simulink model "prueba_dynamixel"  (R2020b)
settings: Solver=VariableStepAuto  StartTime=0.0  StopTime=10.0  RelTol=1e-3
values from neighbouring files (symbols this model uses):
  ADDR_MX_GOAL_POSITION = 30    [variables_dynamixel.m]
  ADDR_MX_PRESENT_POSITION = 36    [variables_dynamixel.m]
  ADDR_MX_TORQUE_ENABLE = 24    [variables_dynamixel.m]
  baud_rate = 57600    [variables_dynamixel.m]
  dynamixel_id = 1    [variables_dynamixel.m]
  protocol_version = 1    [variables_dynamixel.m]
settings Model: Creator=johnc  LastModifiedBy=johnc

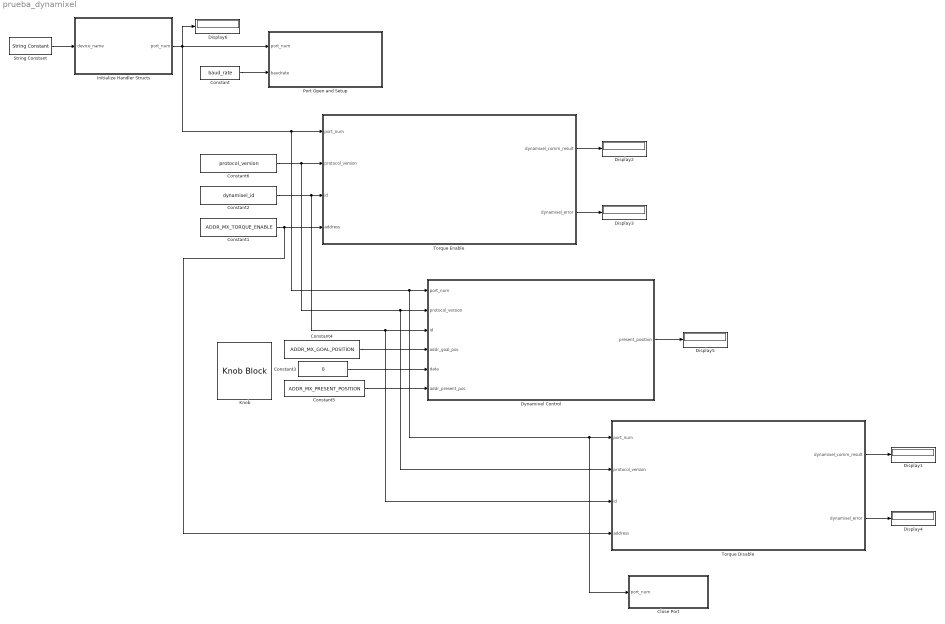
== system prueba_dynamixel ==
  Close Port : MATLAB Function  TreatAsAtomicUnit=on
  Constant : Constant  Value=baud_rate
  Constant1 : Constant  Value=ADDR_MX_TORQUE_ENABLE
  Constant2 : Constant  Value=dynamixel_id
  Constant3 : Constant  Value=0
  Constant4 : Constant  Value=ADDR_MX_GOAL_POSITION
  Constant5 : Constant  Value=ADDR_MX_PRESENT_POSITION
  Constant6 : Constant  Value=protocol_version
  Display{1..6} (6 alike) : Display
  Dynamixel Control : Subsystem
  Initialize Handler Structs : Subsystem
  Knob : KnobBlock  ScaleMax=1023
  Port Open and Setup : Subsystem
  String Constant : StringConstant  String=device_name
  Torque Disable : Subsystem
  Torque Enable : Subsystem
  wires:
  Torque Enable/1(dynamixel_comm_result) -> Display2/1
  Torque Enable/2(dynamixel_error) -> Display3/1
  String Constant/1 -> Initialize Handler Structs/1(device_name)
  Initialize Handler Structs/1(port_num) -> Close Port/1(port_num), Torque Disable/1(port_num), Dynamixel Control/1(port_num), Torque Enable/1(port_num), Display6/1, Port Open and Setup/1(port_num)
  Constant/1 -> Port Open and Setup/2(baudrate)
  Constant1/1 -> Torque Enable/4(address), Torque Disable/4(address)
  Constant2/1 -> Torque Disable/3(id), Dynamixel Control/3(id), Torque Enable/3(id)
  Torque Disable/1(dynamixel_comm_result) -> Display1/1
  Torque Disable/2(dynamixel_error) -> Display4/1
  Dynamixel Control/1(present_position) -> Display5/1
  Constant3/1 -> Dynamixel Control/5(data)
  Constant5/1 -> Dynamixel Control/6(addr_present_pos)
  Constant4/1 -> Dynamixel Control/4(addr_goal_pos)
  Constant6/1 -> Torque Disable/2(protocol_version), Dynamixel Control/2(protocol_version), Torque Enable/2(protocol_version)

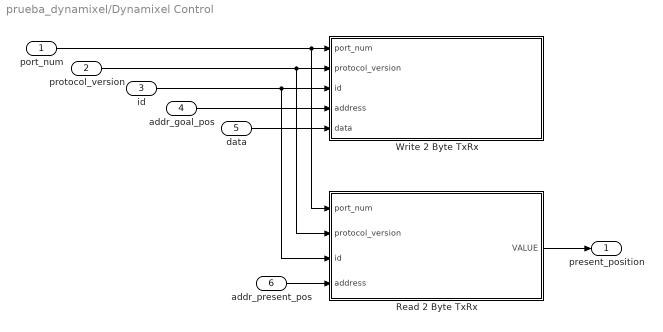
== system prueba_dynamixel/Dynamixel Control ==
  port_num : Inport
  protocol_version : Inport  Port=2
  id : Inport  Port=3
  addr_goal_pos : Inport  Port=4
  data : Inport  Port=5
  addr_present_pos : Inport  Port=6
  Read 2 Byte TxRx : MATLAB Function  TreatAsAtomicUnit=on
  Write 2 Byte TxRx : MATLAB Function  TreatAsAtomicUnit=on
  present_position : Outport
  wires:
  addr_goal_pos/1 -> Write 2 Byte TxRx/4(address)
  data/1 -> Write 2 Byte TxRx/5(data)
  protocol_version/1 -> Write 2 Byte TxRx/2(protocol_version), Read 2 Byte TxRx/2(protocol_version)
  Read 2 Byte TxRx/1(VALUE) -> present_position/1
  port_num/1 -> Write 2 Byte TxRx/1(port_num), Read 2 Byte TxRx/1(port_num)
  id/1 -> Write 2 Byte TxRx/3(id), Read 2 Byte TxRx/3(id)
  addr_present_pos/1 -> Read 2 Byte TxRx/4(address)

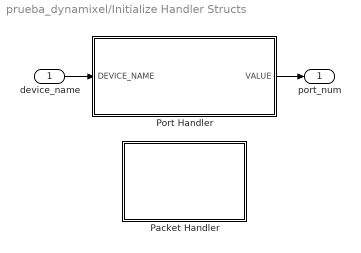
== system prueba_dynamixel/Initialize Handler Structs ==
  device_name : Inport
  Packet Handler : MATLAB Function  TreatAsAtomicUnit=on
  Port Handler : MATLAB Function  TreatAsAtomicUnit=on
  port_num : Outport
  wires:
  device_name/1 -> Port Handler/1(DEVICE_NAME)
  Port Handler/1(VALUE) -> port_num/1

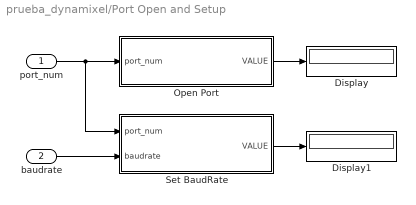
== system prueba_dynamixel/Port Open and Setup ==
  port_num : Inport
  baudrate : Inport  Port=2
  Display : Display
  Display1 : Display
  Open Port : MATLAB Function  TreatAsAtomicUnit=on
  Set BaudRate : MATLAB Function  TreatAsAtomicUnit=on
  wires:
  port_num/1 -> Set BaudRate/1(port_num), Open Port/1(port_num)
  baudrate/1 -> Set BaudRate/2(baudrate)
  Set BaudRate/1(VALUE) -> Display1/1
  Open Port/1(VALUE) -> Display/1

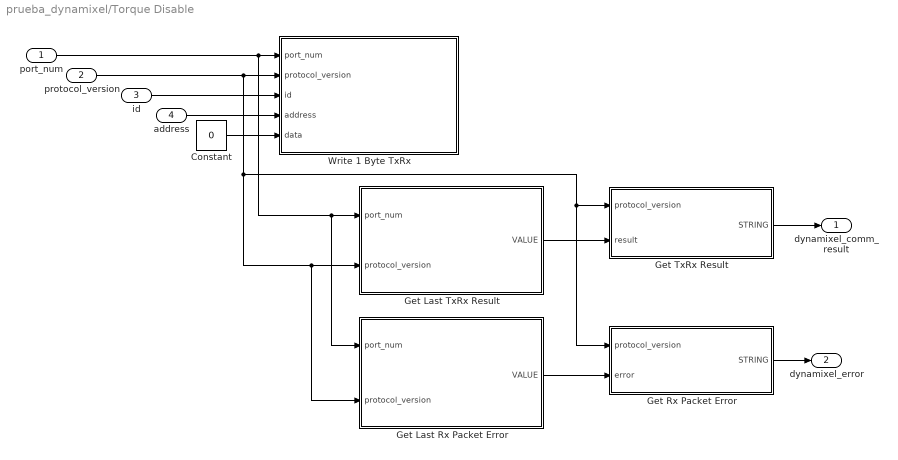
== system prueba_dynamixel/Torque Disable ==
  port_num : Inport
  protocol_version : Inport  Port=2
  id : Inport  Port=3
  address : Inport  Port=4
  Constant : Constant  Value=0
  Get Last Rx Packet Error : MATLAB Function  TreatAsAtomicUnit=on
  Get Last TxRx Result : MATLAB Function  TreatAsAtomicUnit=on
  Get Rx Packet Error : MATLAB Function  TreatAsAtomicUnit=on
  Get TxRx Result : MATLAB Function  TreatAsAtomicUnit=on
  Write 1 Byte TxRx : MATLAB Function  TreatAsAtomicUnit=on
  dynamixel_comm_result : Outport
  dynamixel_error : Outport  Port=2
  wires:
  Constant/1 -> Write 1 Byte TxRx/5(data)
  id/1 -> Write 1 Byte TxRx/3(id)
  Get Last Rx Packet Error/1(VALUE) -> Get Rx Packet Error/2(error)
  Get Last TxRx Result/1(VALUE) -> Get TxRx Result/2(result)
  address/1 -> Write 1 Byte TxRx/4(address)
  port_num/1 -> Get Last Rx Packet Error/1(port_num), Get Last TxRx Result/1(port_num), Write 1 Byte TxRx/1(port_num)
  Get TxRx Result/1(STRING) -> dynamixel_comm_result/1
  protocol_version/1 -> Get Last Rx Packet Error/2(protocol_version), Get Last TxRx Result/2(protocol_version), Get Rx Packet Error/1(protocol_version), Get TxRx Result/1(protocol_version), Write 1 Byte TxRx/2(protocol_version)
  Get Rx Packet Error/1(STRING) -> dynamixel_error/1

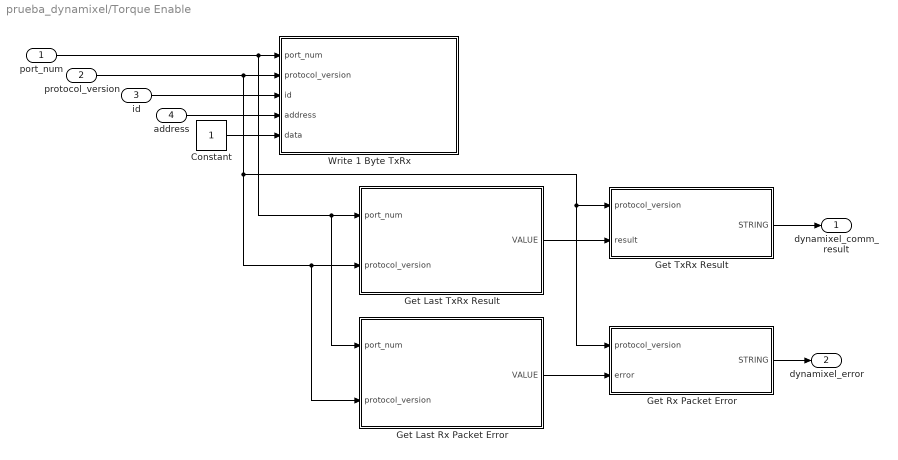
== system prueba_dynamixel/Torque Enable ==
  port_num : Inport
  protocol_version : Inport  Port=2
  id : Inport  Port=3
  address : Inport  Port=4
  Constant : Constant
  Get Last Rx Packet Error : MATLAB Function  TreatAsAtomicUnit=on
  Get Last TxRx Result : MATLAB Function  TreatAsAtomicUnit=on
  Get Rx Packet Error : MATLAB Function  TreatAsAtomicUnit=on
  Get TxRx Result : MATLAB Function  TreatAsAtomicUnit=on
  Write 1 Byte TxRx : MATLAB Function  TreatAsAtomicUnit=on
  dynamixel_comm_result : Outport
  dynamixel_error : Outport  Port=2
  wires:
  Constant/1 -> Write 1 Byte TxRx/5(data)
  id/1 -> Write 1 Byte TxRx/3(id)
  Get Last Rx Packet Error/1(VALUE) -> Get Rx Packet Error/2(error)
  Get Last TxRx Result/1(VALUE) -> Get TxRx Result/2(result)
  address/1 -> Write 1 Byte TxRx/4(address)
  port_num/1 -> Get Last Rx Packet Error/1(port_num), Get Last TxRx Result/1(port_num), Write 1 Byte TxRx/1(port_num)
  Get TxRx Result/1(STRING) -> dynamixel_comm_result/1
  protocol_version/1 -> Get Last Rx Packet Error/2(protocol_version), Get Last TxRx Result/2(protocol_version), Get Rx Packet Error/1(protocol_version), Get TxRx Result/1(protocol_version), Write 1 Byte TxRx/2(protocol_version)
  Get Rx Packet Error/1(STRING) -> dynamixel_error/1

== matlab function prueba_dynamixel/Torque Disable/Get TxRx Result ==
  data: protocol_version input; STRING output; result input
function STRING  = getTxRxResult( protocol_version, result )

lib_name = '';

if strcmp(computer, 'PCWIN')
  lib_name = 'dxl_x86_c';
elseif strcmp(computer, 'PCWIN64')
  lib_name = 'dxl_x64_c';
elseif strcmp(computer, 'GLNX86')
  lib_name = 'libdxl_x86_c';
elseif strcmp(computer, 'GLNXA64')
  lib_name = 'libdxl_x64_c';
elseif strcmp(computer, 'MACI64')
  lib_name = 'libdxl_mac_c';
end

coder.extrinsic('getTxRxResult');
temp = int32(result);
temp1 = int32(protocol_version);
temp2 = string(STRING);

end

== matlab function prueba_dynamixel/Torque Disable/Write 1 Byte TxRx ==
  data: port_num input; protocol_version input; id input; address input; data input
function write1ByteTxRx(port_num, protocol_version, id, address, data)

lib_name = '';

if strcmp(computer, 'PCWIN')
  lib_name = 'dxl_x86_c';
elseif strcmp(computer, 'PCWIN64')
  lib_name = 'dxl_x64_c';
elseif strcmp(computer, 'GLNX86')
  lib_name = 'libdxl_x86_c';
elseif strcmp(computer, 'GLNXA64')
  lib_name = 'libdxl_x64_c';
elseif strcmp(computer, 'MACI64')
  lib_name = 'libdxl_mac_c';
end

coder.extrinsic('write1ByteTxRx');
temp1 = uint8(data);
temp2 = uint16(address);
temp3 = uint8(id);
temp4 = int32(protocol_version);
temp5 = int32(port_num);

end

== matlab function prueba_dynamixel/Initialize Handler Structs/Port Handler ==
  data: DEVICE_NAME input; VALUE output
function VALUE  = portHandler( DEVICE_NAME )

lib_name = '';

if strcmp(computer, 'PCWIN')
  lib_name = 'dxl_x86_c';
elseif strcmp(computer, 'PCWIN64')
  lib_name = 'dxl_x64_c';
elseif strcmp(computer, 'GLNX86')
  lib_name = 'libdxl_x86_c';
elseif strcmp(computer, 'GLNXA64')
  lib_name = 'libdxl_x64_c';
elseif strcmp(computer, 'MACI64')
  lib_name = 'libdxl_mac_c';
end

coder.extrinsic('portHandler');
temp = string(DEVICE_NAME);
temp1 = int32(VALUE);

end

== matlab function prueba_dynamixel/Close Port ==
  data: port_num input
function closePort(port_num)

lib_name = '';

if strcmp(computer, 'PCWIN')
  lib_name = 'dxl_x86_c';
elseif strcmp(computer, 'PCWIN64')
  lib_name = 'dxl_x64_c';
elseif strcmp(computer, 'GLNX86')
  lib_name = 'libdxl_x86_c';
elseif strcmp(computer, 'GLNXA64')
  lib_name = 'libdxl_x64_c';
elseif strcmp(computer, 'MACI64')
  lib_name = 'libdxl_mac_c';
end

coder.extrinsic('closePort');
temp = int32(port_num);

end

== matlab function prueba_dynamixel/Dynamixel Control/Write 2 Byte TxRx ==
  data: port_num input; protocol_version input; id input; address input; data input
function write2ByteTxRx(port_num, protocol_version, id, address, data)

lib_name = '';

if strcmp(computer, 'PCWIN')
  lib_name = 'dxl_x86_c';
elseif strcmp(computer, 'PCWIN64')
  lib_name = 'dxl_x64_c';
elseif strcmp(computer, 'GLNX86')
  lib_name = 'libdxl_x86_c';
elseif strcmp(computer, 'GLNXA64')
  lib_name = 'libdxl_x64_c';
elseif strcmp(computer, 'MACI64')
  lib_name = 'libdxl_mac_c';
end

coder.extrinsic('write2ByteTxRx');
temp = uint16(data);
temp1 = uint16(address);
temp2 = uint8(id);
temp3 = int32(protocol_version);
temp4 = int32(port_num);

end

== matlab function prueba_dynamixel/Dynamixel Control/Read 2 Byte TxRx ==
  data: port_num input; VALUE output; protocol_version input; id input; address input
function VALUE = read2ByteTxRx( port_num, protocol_version, id, address )

lib_name = '';

if strcmp(computer, 'PCWIN')
  lib_name = 'dxl_x86_c';
elseif strcmp(computer, 'PCWIN64')
  lib_name = 'dxl_x64_c';
elseif strcmp(computer, 'GLNX86')
  lib_name = 'libdxl_x86_c';
elseif strcmp(computer, 'GLNXA64')
  lib_name = 'libdxl_x64_c';
elseif strcmp(computer, 'MACI64')
  lib_name = 'libdxl_mac_c';
end

coder.extrinsic('read2ByteTxRx');
temp = uint16(address);
temp1 = uint8(id);
temp2 = int32(protocol_version);
temp3 = int32(port_num);
temp4 = uint16(VALUE);

end

== matlab function prueba_dynamixel/Initialize Handler Structs/Packet Handler ==
function packetHandler

lib_name = '';

if strcmp(computer, 'PCWIN')
  lib_name = 'dxl_x86_c';
elseif strcmp(computer, 'PCWIN64')
  lib_name = 'dxl_x64_c';
elseif strcmp(computer, 'GLNX86')
  lib_name = 'libdxl_x86_c';
elseif strcmp(computer, 'GLNXA64')
  lib_name = 'libdxl_x64_c';
elseif strcmp(computer, 'MACI64')
  lib_name = 'libdxl_mac_c';
end

coder.extrinsic('packetHandler');

end

== matlab function prueba_dynamixel/Port Open and Setup/Open Port ==
  data: port_num input int32; VALUE output uint8
function VALUE  = openPort( port_num )

lib_name = '';

if strcmp(computer, 'PCWIN')
  lib_name = 'dxl_x86_c';
elseif strcmp(computer, 'PCWIN64')
  lib_name = 'dxl_x64_c';
elseif strcmp(computer, 'GLNX86')
  lib_name = 'libdxl_x86_c';
elseif strcmp(computer, 'GLNXA64')
  lib_name = 'libdxl_x64_c';
elseif strcmp(computer, 'MACI64')
  lib_name = 'libdxl_mac_c';
end

coder.extrinsic('openPort');
temp1 = int32(port_num);
temp2 = uint8(VALUE);

end

== matlab function prueba_dynamixel/Port Open and Setup/Set BaudRate ==
  data: port_num input; VALUE output; baudrate input
function VALUE  = setBaudRate( port_num, baudrate )

lib_name = '';

if strcmp(computer, 'PCWIN')
  lib_name = 'dxl_x86_c';
elseif strcmp(computer, 'PCWIN64')
  lib_name = 'dxl_x64_c';
elseif strcmp(computer, 'GLNX86')
  lib_name = 'libdxl_x86_c';
elseif strcmp(computer, 'GLNXA64')
  lib_name = 'libdxl_x64_c';
elseif strcmp(computer, 'MACI64')
  lib_name = 'libdxl_mac_c';
end

coder.extrinsic('setBaudRate');
temp = int32(baudrate);
temp1 = int32(port_num);
temp2 = uint8(VALUE);

end

== matlab function prueba_dynamixel/Torque Enable/Write 1 Byte TxRx ==
  data: port_num input; protocol_version input; id input; address input; data input
function write1ByteTxRx(port_num, protocol_version, id, address, data)

lib_name = '';

if strcmp(computer, 'PCWIN')
  lib_name = 'dxl_x86_c';
elseif strcmp(computer, 'PCWIN64')
  lib_name = 'dxl_x64_c';
elseif strcmp(computer, 'GLNX86')
  lib_name = 'libdxl_x86_c';
elseif strcmp(computer, 'GLNXA64')
  lib_name = 'libdxl_x64_c';
elseif strcmp(computer, 'MACI64')
  lib_name = 'libdxl_mac_c';
end

coder.extrinsic('write1ByteTxRx');
temp1 = uint8(data);
temp2 = uint16(address);
temp3 = uint8(id);
temp4 = int32(protocol_version);
temp5 = int32(port_num);

end

== matlab function prueba_dynamixel/Torque Enable/Get Last TxRx Result ==
  data: port_num input; VALUE output; protocol_version input
function VALUE  = getLastTxRxResult( port_num, protocol_version )

lib_name = '';

if strcmp(computer, 'PCWIN')
  lib_name = 'dxl_x86_c';
elseif strcmp(computer, 'PCWIN64')
  lib_name = 'dxl_x64_c';
elseif strcmp(computer, 'GLNX86')
  lib_name = 'libdxl_x86_c';
elseif strcmp(computer, 'GLNXA64')
  lib_name = 'libdxl_x64_c';
elseif strcmp(computer, 'MACI64')
  lib_name = 'libdxl_mac_c';
end

coder.extrinsic('getLastTxRxResult');
temp = int32(protocol_version);
temp1 = int32(port_num);
temp2 = int32(VALUE);

end

== matlab function prueba_dynamixel/Torque Enable/Get Last Rx Packet Error ==
  data: port_num input; VALUE output; protocol_version input
function VALUE  = getLastRxPacketError( port_num, protocol_version )

lib_name = '';

if strcmp(computer, 'PCWIN')
  lib_name = 'dxl_x86_c';
elseif strcmp(computer, 'PCWIN64')
  lib_name = 'dxl_x64_c';
elseif strcmp(computer, 'GLNX86')
  lib_name = 'libdxl_x86_c';
elseif strcmp(computer, 'GLNXA64')
  lib_name = 'libdxl_x64_c';
elseif strcmp(computer, 'MACI64')
  lib_name = 'libdxl_mac_c';
end

coder.extrinsic('getLastRxPacketError');
temp = int32(protocol_version);
temp1 = int32(port_num);
temp2 = uint8(VALUE);

end

== matlab function prueba_dynamixel/Torque Enable/Get TxRx Result ==
  data: protocol_version input; STRING output; result input
function STRING  = getTxRxResult( protocol_version, result )

lib_name = '';

if strcmp(computer, 'PCWIN')
  lib_name = 'dxl_x86_c';
elseif strcmp(computer, 'PCWIN64')
  lib_name = 'dxl_x64_c';
elseif strcmp(computer, 'GLNX86')
  lib_name = 'libdxl_x86_c';
elseif strcmp(computer, 'GLNXA64')
  lib_name = 'libdxl_x64_c';
elseif strcmp(computer, 'MACI64')
  lib_name = 'libdxl_mac_c';
end

coder.extrinsic('getTxRxResult');
temp = int32(result);
temp1 = int32(protocol_version);
temp2 = string(STRING);

end

== matlab function prueba_dynamixel/Torque Enable/Get Rx Packet Error ==
  data: protocol_version input; STRING output; error input
function STRING  = getRxPacketError( protocol_version, error )

lib_name = '';

if strcmp(computer, 'PCWIN')
  lib_name = 'dxl_x86_c';
elseif strcmp(computer, 'PCWIN64')
  lib_name = 'dxl_x64_c';
elseif strcmp(computer, 'GLNX86')
  lib_name = 'libdxl_x86_c';
elseif strcmp(computer, 'GLNXA64')
  lib_name = 'libdxl_x64_c';
elseif strcmp(computer, 'MACI64')
  lib_name = 'libdxl_mac_c';
end

coder.extrinsic('getRxPacketError');
temp = uint8(error);
temp1 = int32(protocol_version);
temp2 = string(STRING);

end

== matlab function prueba_dynamixel/Torque Disable/Get Last Rx Packet Error ==
  data: port_num input; VALUE output; protocol_version input
function VALUE  = getLastRxPacketError( port_num, protocol_version )

lib_name = '';

if strcmp(computer, 'PCWIN')
  lib_name = 'dxl_x86_c';
elseif strcmp(computer, 'PCWIN64')
  lib_name = 'dxl_x64_c';
elseif strcmp(computer, 'GLNX86')
  lib_name = 'libdxl_x86_c';
elseif strcmp(computer, 'GLNXA64')
  lib_name = 'libdxl_x64_c';
elseif strcmp(computer, 'MACI64')
  lib_name = 'libdxl_mac_c';
end

coder.extrinsic('getLastRxPacketError');
temp = int32(protocol_version);
temp1 = int32(port_num);
temp2 = uint8(VALUE);

end

== matlab function prueba_dynamixel/Torque Disable/Get Last TxRx Result ==
  data: port_num input; VALUE output; protocol_version input
function VALUE  = getLastTxRxResult( port_num, protocol_version )

lib_name = '';

if strcmp(computer, 'PCWIN')
  lib_name = 'dxl_x86_c';
elseif strcmp(computer, 'PCWIN64')
  lib_name = 'dxl_x64_c';
elseif strcmp(computer, 'GLNX86')
  lib_name = 'libdxl_x86_c';
elseif strcmp(computer, 'GLNXA64')
  lib_name = 'libdxl_x64_c';
elseif strcmp(computer, 'MACI64')
  lib_name = 'libdxl_mac_c';
end

coder.extrinsic('getLastTxRxResult');
temp = int32(protocol_version);
temp1 = int32(port_num);
temp2 = int32(VALUE);

end

== matlab function prueba_dynamixel/Torque Disable/Get Rx Packet Error ==
  data: protocol_version input; STRING output; error input
function STRING  = getRxPacketError( protocol_version, error )

lib_name = '';

if strcmp(computer, 'PCWIN')
  lib_name = 'dxl_x86_c';
elseif strcmp(computer, 'PCWIN64')
  lib_name = 'dxl_x64_c';
elseif strcmp(computer, 'GLNX86')
  lib_name = 'libdxl_x86_c';
elseif strcmp(computer, 'GLNXA64')
  lib_name = 'libdxl_x64_c';
elseif strcmp(computer, 'MACI64')
  lib_name = 'libdxl_mac_c';
end

coder.extrinsic('getRxPacketError');
temp = uint8(error);
temp1 = int32(protocol_version);
temp2 = string(STRING);

end
